simulink model "PID_controller"  (R2021a)
settings: Solver=FixedStepAuto  StartTime=0.0  StopTime=20  FixedStep=0.001  RelTol=1e-3
settings Model: Creator=Davie  LastModifiedBy=Davie

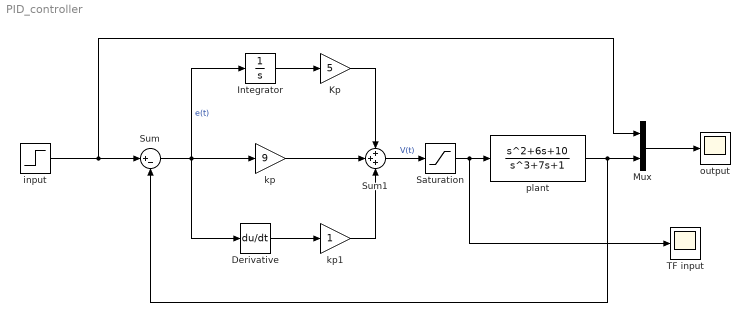
== system PID_controller ==
  Derivative : Derivative
  Integrator : Integrator
  Kp : Gain  Gain=5
  Mux : Mux  Inputs=2
  Saturation : Saturate  UpperLimit=2  LowerLimit=-2
  Sum : Sum  Inputs=|+-
  Sum1 : Sum  Inputs=+++
  TF input : Scope
  input : Step  SampleTime=0
  kp : Gain  Gain=9
  kp1 : Gain
  output : Scope
  plant : TransferFcn  Numerator=[1 6 10]  Denominator=[1 0 7 1]
  wires:
  input/1 -> Mux/1, Sum/1
  Sum/1 -> Derivative/1, Integrator/1, kp/1  "e(t)"
  plant/1 -> Mux/2, Sum/2
  kp/1 -> Sum1/2
  Mux/1 -> output/1
  Integrator/1 -> Kp/1
  Sum1/1 -> Saturation/1  "V(t)"
  Kp/1 -> Sum1/1
  Derivative/1 -> kp1/1
  kp1/1 -> Sum1/3
  Saturation/1 -> TF input/1, plant/1
